simulink model "Aenea_model"  (R2020b)
settings: Solver=FixedStepDiscrete  StartTime=0.0  StopTime=10.0  FixedStep=0.02  RelTol=1e-3
undefined symbols (not defined in the file): attuatore_Amax, attuatore_Amin, attuatore_Emax, attuatore_Emin, attuatore_Rmax, attuatore_Rmin, attuatore_Tmax, attuatore_Tmin, bias, DiscIntNeverNeededParam, interventoA_05, interventoA_1, interventoE_05, interventoE_1, interventoT, inv_A, inv_comp_h, inv_E, inv_R, inv_T, K_AW_B_AP_quota, K_AW_B_becc, K_AW_B_imb, K_AW_B_roll, K_imb_inv, Kd_h_app, Kd_h_flare, Ki_AP_quota_select, Ki_AP_rotta, Ki_AP_vel, Ki_becch, Ki_h_app, Ki_h_cruise, Ki_h_flare, Ki_roll, Kp_AP_quota_hold_h, Kp_AP_quota_hold_l, Kp_AP_quota_select, Kp_AP_rotta, Kp_AP_vel, Kp_becch, Kp_comp_h, Kp_h_app_max, Kp_h_app_min, Kp_h_cruise, Kp_h_flare, Kp_imb, Kp_p, Kp_q, Kp_roll, Kp_Rotta_ATO, Newton, phi_max, phi_min, Q1B, R1B, Raphson, safe_phi, safe_V, Sensor_Offsets ... (+12)
libraries: simulink_extras x37, pid_lib x8, dspsigops x4, arduinolib x3, svdutilitieslib x3, simulink x2, aerolibtransform2sys x2, aerolibtransform2 x2, aerosimlib x2, cstblocks x1
(part 3 of 7)

== system Aenea_model/RADIOCOMANDO/AILERON1 ==
  pwm_aileron_max : Inport
  In1 : Inport  Port=2
  pwm_aileron_min : Inport  Port=3
  Constant8 : Constant  Value=phi_max  OutDataTypeStr=double  SampleTime=-1
  Constant9 : Constant  Value=phi_min  OutDataTypeStr=double  SampleTime=-1
  Divide : Product  Inputs=*/
  Gain : Gain  Gain=-1
  Multiply : Product
  Saturation : Saturate  UpperLimit=phi_max  LowerLimit=phi_min
  Sum : Sum  Inputs=|+-
  Sum1 : Sum  Inputs=|+-
  Sum2 : Sum  Inputs=|+-
  Sum3 : Sum  Inputs=|++
  Out1 : Outport  VectorParamsAs1DForOutWhenUnconnected=off
  wires:
  Divide/1 -> Multiply/1
  Sum/1 -> Divide/1
  In1/1 -> Sum/1
  Constant8/1 -> Sum2/1
  pwm_aileron_min/1 -> Sum1/2, Sum/2
  pwm_aileron_max/1 -> Sum1/1
  Multiply/1 -> Sum3/1
  Sum2/1 -> Multiply/2
  Constant9/1 -> Sum3/2, Sum2/2
  Sum1/1 -> Divide/2
  Sum3/1 -> Gain/1
  Gain/1 -> Saturation/1
  Saturation/1 -> Out1/1

== system Aenea_model/RADIOCOMANDO/ELEVATOR ==
  pwm_elevator_max : Inport
  In1 : Inport  Port=2
  pwm_elevator_min : Inport  Port=3
  Constant8 : Constant  Value=attuatore_Emax  OutDataTypeStr=double  SampleTime=-1
  Constant9 : Constant  Value=attuatore_Emin  OutDataTypeStr=double  SampleTime=-1
  Divide : Product  Inputs=*/
  Multiply : Product
  Sum : Sum  Inputs=|+-
  Sum1 : Sum  Inputs=|+-
  Sum2 : Sum  Inputs=|+-
  Sum3 : Sum  Inputs=|++
  Out1 : Outport  VectorParamsAs1DForOutWhenUnconnected=off
  wires:
  Sum3/1 -> Out1/1
  Multiply/1 -> Sum3/1
  Constant9/1 -> Sum3/2, Sum2/2
  Sum1/1 -> Divide/2
  Sum2/1 -> Multiply/2
  pwm_elevator_min/1 -> Sum1/2, Sum/2
  Constant8/1 -> Sum2/1
  pwm_elevator_max/1 -> Sum1/1
  Divide/1 -> Multiply/1
  In1/1 -> Sum/1
  Sum/1 -> Divide/1

== system Aenea_model/RADIOCOMANDO/ELEVATOR1 ==
  pwm_elevator_max : Inport
  In1 : Inport  Port=2
  pwm_elevator_min : Inport  Port=3
  Constant8 : Constant  Value=theta_max  OutDataTypeStr=double  SampleTime=-1
  Constant9 : Constant  Value=theta_min  OutDataTypeStr=double  SampleTime=-1
  Divide : Product  Inputs=*/
  Gain : Gain
  Multiply : Product
  Saturation : Saturate  UpperLimit=theta_max  LowerLimit=theta_min
  Sum : Sum  Inputs=|+-
  Sum1 : Sum  Inputs=|+-
  Sum2 : Sum  Inputs=|+-
  Sum3 : Sum  Inputs=|++
  Out1 : Outport  VectorParamsAs1DForOutWhenUnconnected=off
  wires:
  Sum3/1 -> Gain/1
  Multiply/1 -> Sum3/1
  Constant9/1 -> Sum3/2, Sum2/2
  Sum1/1 -> Divide/2
  Sum2/1 -> Multiply/2
  pwm_elevator_min/1 -> Sum1/2, Sum/2
  Constant8/1 -> Sum2/1
  pwm_elevator_max/1 -> Sum1/1
  Divide/1 -> Multiply/1
  In1/1 -> Sum/1
  Sum/1 -> Divide/1
  Gain/1 -> Saturation/1
  Saturation/1 -> Out1/1

== system Aenea_model/RADIOCOMANDO/RUDDER ==
  pwm_rudder_max : Inport
  In1 : Inport  Port=2
  pwm_rudder_min : Inport  Port=3
  Constant8 : Constant  Value=attuatore_Rmax  OutDataTypeStr=double  SampleTime=-1
  Constant9 : Constant  Value=attuatore_Rmin  OutDataTypeStr=double  SampleTime=-1
  Divide : Product  Inputs=*/
  Multiply : Product
  Sum1 : Sum  Inputs=|+-
  Sum2 : Sum  Inputs=|+-
  Sum3 : Sum  Inputs=|+-
  Sum4 : Sum  Inputs=|++
  Out1 : Outport  VectorParamsAs1DForOutWhenUnconnected=off
  wires:
  Divide/1 -> Multiply/1
  Sum2/1 -> Divide/2
  pwm_rudder_min/1 -> Sum1/2, Sum2/2
  Sum3/1 -> Multiply/2
  Multiply/1 -> Sum4/1
  Constant9/1 -> Sum4/2, Sum3/2
  Sum1/1 -> Divide/1
  Constant8/1 -> Sum3/1
  pwm_rudder_max/1 -> Sum2/1
  Sum4/1 -> Out1/1
  In1/1 -> Sum1/1

== system Aenea_model/RADIOCOMANDO/THROTTLE ==
  pwm_throttle_max : Inport
  In1 : Inport  Port=2
  pwm_throttle_min : Inport  Port=3
  Divide2 : Product  Inputs=*/
  Multiply1 : Product
  Sum2 : Sum  Inputs=|+-
  Sum3 : Sum  Inputs=|+-
  Sum4 : Sum  Inputs=|+-
  Sum5 : Sum  Inputs=|++
  manetta_massima : Constant  Value=attuatore_Tmax  OutDataTypeStr=double  SampleTime=-1
  manetta_minima : Constant  Value=attuatore_Tmin  OutDataTypeStr=double  SampleTime=-1
  Out1 : Outport  VectorParamsAs1DForOutWhenUnconnected=off
  wires:
  Sum4/1 -> Multiply1/2
  Divide2/1 -> Multiply1/1
  pwm_throttle_max/1 -> Sum3/1
  Sum3/1 -> Divide2/2
  Sum2/1 -> Divide2/1
  manetta_minima/1 -> Sum4/2, Sum5/2
  pwm_throttle_min/1 -> Sum3/2, Sum2/2
  In1/1 -> Sum2/1
  Multiply1/1 -> Sum5/1
  Sum5/1 -> Out1/1
  manetta_massima/1 -> Sum4/1

== system Aenea_model/Servi/AILERON1 ==
  pwm_aileron_max : Inport
  In1 : Inport  Port=2
  pwm-aileron_min : Inport  Port=3
  Constant : Constant  Value=attuatore_Amax  SampleTime=t_AP
  Constant1 : Constant  Value=attuatore_Amin  SampleTime=t_AP
  Divide : Product  Inputs=*/
  Multiply : Product
  Sum : Sum  Inputs=|+-
  Sum1 : Sum  Inputs=|+-
  Sum2 : Sum  Inputs=|+-
  Sum3 : Sum  Inputs=|++
  Out1 : Outport  VectorParamsAs1DForOutWhenUnconnected=off
  wires:
  Sum/1 -> Divide/1
  Constant1/1 -> Sum1/2, Sum/2
  In1/1 -> Sum/1
  Divide/1 -> Multiply/1
  Sum2/1 -> Multiply/2
  pwm-aileron_min/1 -> Sum2/2, Sum3/2
  Multiply/1 -> Sum3/1
  Sum3/1 -> Out1/1
  pwm_aileron_max/1 -> Sum2/1
  Constant/1 -> Sum1/1
  Sum1/1 -> Divide/2

== system Aenea_model/Servi/RUDDER6 ==
  pwm_rudder_max : Inport
  In1 : Inport  Port=2
  "pwm_rudder_min " : Inport  Port=3
  Constant : Constant  Value=attuatore_Rmax  SampleTime=t_AP
  Constant1 : Constant  Value=attuatore_Rmin  SampleTime=t_AP
  Divide : Product  Inputs=*/
  Multiply : Product
  Sum : Sum  Inputs=|+-
  Sum1 : Sum  Inputs=|+-
  Sum2 : Sum  Inputs=|+-
  Sum3 : Sum  Inputs=|++
  Out1 : Outport  VectorParamsAs1DForOutWhenUnconnected=off
  wires:
  Sum/1 -> Divide/1
  Constant1/1 -> Sum1/2, Sum/2
  In1/1 -> Sum/1
  Divide/1 -> Multiply/1
  Sum2/1 -> Multiply/2
  "pwm_rudder_min "/1 -> Sum2/2, Sum3/2
  Multiply/1 -> Sum3/1
  Sum3/1 -> Out1/1
  pwm_rudder_max/1 -> Sum2/1
  Constant/1 -> Sum1/1
  Sum1/1 -> Divide/2

== system Aenea_model/Servi/THROTTLE1 ==
  pwm_throttle_max : Inport
  In1 : Inport  Port=2
  pwm_throttle_min : Inport  Port=3
  Multiply : Product
  Sum : Sum  Inputs=|++  AccumDataTypeStr=int16  OutDataTypeStr=int16
  Sum1 : Sum  Inputs=|+-
  Out1 : Outport  VectorParamsAs1DForOutWhenUnconnected=off
  wires:
  pwm_throttle_min/1 -> Sum/2, Sum1/2
  Sum/1 -> Out1/1
  Multiply/1 -> Sum/1
  pwm_throttle_max/1 -> Sum1/1
  Sum1/1 -> Multiply/2
  In1/1 -> Multiply/1

== system Aenea_model/Servi/elevator ==
  pwm_elevator_max : Inport
  In1 : Inport  Port=2
  pwm_elevator_min : Inport  Port=3
  Constant : Constant  Value=attuatore_Emax  SampleTime=t_AP
  Constant1 : Constant  Value=attuatore_Emin  SampleTime=t_AP
  Divide : Product  Inputs=*/
  Multiply : Product
  Sum : Sum  Inputs=|+-
  Sum1 : Sum  Inputs=|+-
  Sum2 : Sum  Inputs=|+-
  Sum3 : Sum  Inputs=|++
  Out1 : Outport  VectorParamsAs1DForOutWhenUnconnected=off
  wires:
  In1/1 -> Sum/1
  Constant1/1 -> Sum1/2, Sum/2
  Constant/1 -> Sum1/1
  Sum/1 -> Divide/1
  Sum1/1 -> Divide/2
  Divide/1 -> Multiply/1
  pwm_elevator_max/1 -> Sum2/1
  pwm_elevator_min/1 -> Sum2/2, Sum3/2
  Sum2/1 -> Multiply/2
  Multiply/1 -> Sum3/1
  Sum3/1 -> Out1/1

== system Aenea_model/AIR TX/Enable /Chart/sendbyte ==
  note: sostituito con lo stesso blocco della V. R2015a il 29/1/2016
  bt : Inport  OutDataTypeStr=uint8
  n : Inport  Port=2
  f : TriggerPort  TriggerType=function-call  VariantControl=(inherit)
      settings: CopyFcn=Stateflow.SLINSF.SimulinkMan.removeBlockPreDeleteFcn  PreDeleteFcn=Stateflow.SLINSF.SimulinkMan.unsafePredeleteFcn
  Selector : Selector  InputPortWidth=264  IndexOptions=Index vector (port)  Indices=[1 3]  OutputSizes=1
  Serial Transmit : arduinolib/Serial Transmit  Commented=on  portNumber=2  sendmode=write  sendformat=Decimal  floatprecision=2  blockPlatform=arduino
  Terminator : Terminator
  wires:
  Selector/1 -> Terminator/1
  n/1 -> Selector/2
  bt/1 -> Selector/1

== system Aenea_model/AIR TX/If_subsystem/Subsystem ==
  Add : Sum  Inputs=+++
  Add1 : Sum  Inputs=+++
  Add2 : Sum  Inputs=+++
  Constant : Constant  Value=0  SampleTime=0.02
  Constant1 : Constant  Value=0.02  SampleTime=0.02
  Constant2 : Constant  Value=0  SampleTime=t_AP
  Constant3 : Constant  SampleTime=t_AP
  Constant4 : Constant  Value=0  SampleTime=5*t_AP
  Constant5 : Constant  SampleTime=5*t_AP
  Memory : Memory  InitialCondition=-0.02  InheritSampleTime=on
  Memory1 : Memory  InitialCondition=-1  InheritSampleTime=on
  Memory2 : Memory  InitialCondition=-1  InheritSampleTime=on
  Rate Transition : RateTransition  Deterministic=off  OutPortSampleTime=t_AP
  Switch : Switch  Criteria=u2 > Threshold  Threshold=4
  Switch1 : Switch  Criteria=u2 > Threshold  Threshold=9
  H_50 : Outport  VectorParamsAs1DForOutWhenUnconnected=off
  H_10 : Outport  Port=2  VectorParamsAs1DForOutWhenUnconnected=off
  time : Outport  Port=3  VectorParamsAs1DForOutWhenUnconnected=off
  wires:
  Memory1/1 -> Add1/3
  Add2/1 -> Switch1/2, Switch1/3
  Constant4/1 -> Add2/1, Switch1/1
  Constant5/1 -> Add2/2
  Memory2/1 -> Add2/3
  Memory/1 -> Add/3
  Add/1 -> time/1, Memory/1
  Constant/1 -> Add/1
  Constant1/1 -> Add/2
  Constant2/1 -> Add1/1, Switch/1
  Switch/1 -> H_50/1, Memory1/1
  Constant3/1 -> Add1/2
  Add1/1 -> Switch/2, Switch/3
  Switch1/1 -> Rate Transition/1, Memory2/1
  Rate Transition/1 -> H_10/1

== system Aenea_model/AIR TX/Servo/Conversione ==
  Manetta : Inport
  Equilibratore : Inport  Port=2
  Alettoni : Inport  Port=3
  Timone : Inport  Port=4
  Constant2 : Constant  Value=90
  Gain2 : Gain  Gain=100
  Radians to Degrees1 : simulink_extras/Transformations/Radians to Degrees
  Radians to Degrees2 : simulink_extras/Transformations/Radians to Degrees
  Radians to Degrees3 : simulink_extras/Transformations/Radians to Degrees
  Sum : Sum  Inputs=|++
  Sum1 : Sum  Inputs=|++
  Sum2 : Sum  Inputs=|++
  Out1 : Outport  VectorParamsAs1DForOutWhenUnconnected=off
  Out2 : Outport  Port=2  VectorParamsAs1DForOutWhenUnconnected=off
  Out3 : Outport  Port=3  VectorParamsAs1DForOutWhenUnconnected=off
  Out4 : Outport  Port=4  VectorParamsAs1DForOutWhenUnconnected=off
  wires:
  Sum2/1 -> Out4/1
  Timone/1 -> Radians to Degrees3/1
  Sum1/1 -> Out3/1
  Alettoni/1 -> Radians to Degrees2/1
  Sum/1 -> Out2/1
  Equilibratore/1 -> Radians to Degrees1/1
  Gain2/1 -> Out1/1
  Manetta/1 -> Gain2/1
  Constant2/1 -> Sum2/2, Sum1/2, Sum/2
  Radians to Degrees3/1 -> Sum2/1
  Radians to Degrees2/1 -> Sum1/1
  Radians to Degrees1/1 -> Sum/1

== system Aenea_model/AIR TX/VFR/wrapTo360 ==
  In1 : Inport
  Abs : Abs
  Constant2 : Constant  Value=360
  Sum : Sum  Inputs=-+|
  Switch2 : Switch  Criteria=u2 > Threshold
  Out1 : Outport  VectorParamsAs1DForOutWhenUnconnected=off
  wires:
  Sum/1 -> Switch2/3
  Abs/1 -> Sum/1
  Constant2/1 -> Sum/2
  In1/1 -> Switch2/1, Switch2/2, Abs/1
  Switch2/1 -> Out1/1

== system Aenea_model/AUTOPILOTA/AUTOPILOTI1/CONTROLLORE DI QUOTA ==
  Sensori : Inport
  Riferimenti : Inport  Port=2
  Parametri Sistema di Controllo : Inport  Port=3
  Ato : Inport  Port=4
  traking_theta : Inport  Port=5
  Abs : Abs
  Bus Selector : BusSelector  OutputSignals=Kp_AP_quota_hold
  Bus Selector2 : BusSelector  OutputSignals=RC,Alt,Tas,theta
  Bus Selector3 : BusSelector  OutputSignals=QUOTA,RC,landing_selector
  Controllore di RC1 : Subsystem
  Kp : Product  RndMeth=Zero
  SELEZIONE MODALITA' HOLD/SELECT : Stateflow chart  TreatAsAtomicUnit=on
  "Saturazione RC " : Subsystem
  Sum1 : Sum  Inputs=+-
  Switch HOLD/SELECT : MultiPortSwitch  DataPortOrder=Zero-based contiguous  Inputs=2  zeroidx=on
  theta_rif : Outport  VectorParamsAs1DForOutWhenUnconnected=off
  tag scope: RC=global, RC_rif=global, V=global, h=global, h_rif=global, landing_selector=global, parametri_est=global, theta=global
  wires:
  Sensori/1 -> Bus Selector2/1
  Riferimenti/1 -> Bus Selector3/1
  Parametri Sistema di Controllo/1 -> [parametri_est]
  Bus Selector2/1 -> [RC]  "<RC>"
  Bus Selector2/2 -> [h]  "<Alt>"
  Bus Selector2/3 -> [V]  "<Tas>"
  Bus Selector2/4 -> [theta]  "<theta>"
  Bus Selector3/1 -> [h_rif]  "<QUOTA>"
  Bus Selector3/2 -> [RC_rif]  "<RC>"
  [V] -> "Saturazione RC "/1(V)
  Sum1/1 -> Abs/1, Kp/1  "errore_h"
  [h_rif] -> Sum1/1
  [h] -> Sum1/2
  Abs/1 -> SELEZIONE MODALITA' HOLD/SELECT/1(deltah)
  Kp/1 -> Switch HOLD/SELECT/2
  [RC_rif] -> Switch HOLD/SELECT/3
  SELEZIONE MODALITA' HOLD/SELECT/1(mod) -> Switch HOLD/SELECT/1, Controllore di RC1/7(saturation)
  [parametri_est] -> Bus Selector/1
  Bus Selector/1 -> Kp/2  "<Kp_AP_quota_hold>"
  Switch HOLD/SELECT/1 -> "Saturazione RC "/2(RC)
  Bus Selector3/3 -> [landing_selector]  "<landing_selector>"
  [h] -> Controllore di RC1/2(h)
  [h_rif] -> Controllore di RC1/1(h_rif)
  [landing_selector] -> Controllore di RC1/4(landing_selector)
  Ato/1 -> Controllore di RC1/3("Ato ")
  Controllore di RC1/1(theta_rif) -> theta_rif/1
  [RC] -> Controllore di RC1/6(RC)
  "Saturazione RC "/1(RC_verficata) -> Controllore di RC1/5(RC_rif_cruise)
  [RC_rif] -> Controllore di RC1/8("RC_al ")
  traking_theta/1 -> Controllore di RC1/9(traking)
  [V] -> Controllore di RC1/10(tas)

== system Aenea_model/AUTOPILOTA/AUTOPILOTI1/CONTROLLORE DI ROTTA ==
  Riferimenti : Inport
  Sensori : Inport  Port=2
  Parametri Sistema di Controllo : Inport  Port=3
  "switch alettoni " : Inport  Port=4
  track_phi : Inport  Port=5
  Switch_ATO : Inport  Port=6
  ATO : Subsystem
  Bus Selector1 : BusSelector  OutputSignals=ROTTA
  Bus Selector3 : BusSelector  OutputSignals=Kp_AP_rotta,Ki_AP_rotta
  Bus Selector4 : BusSelector  OutputSignals=heading,horiz_speed,Tas,phi,Alt,psi
  Constant : Constant  Value=70
  Constant2 : Constant  Value=Ki_AP_rotta
  PID Controller1 : pid_lib/PID Controller  Controller=PID  Form=Parallel  TimeDomain=Discrete-time  UseExternalTs=off  SampleTime=-1  IntegratorMethod=Forward Euler  FilterMethod=Forward Euler  ControllerParametersSource=external  P=1  I=1  D=0  UseFilter=on  N=100  TunerSelectOption=Transfer Function Based (PID Tuner App)  InitialConditionSource=internal  InitialConditionForIntegrator=0  InitialConditionForFilter=0  DifferentiatorICPrevScaledInput=0  ExternalReset=none  TrackingMode=on  Kt=1  LimitOutput=on  SatLimitsSource=internal  UpperSaturationLimit=0.7854  LowerSaturationLimit=-0.7854  LinearizeAsGain=on  AntiWindupMode=clamping  Kb=0.1  POutMin=[]  POutMax=[]  IOutMin=[]  IOutMax=[]  DOutMin=[]  DOutMax=[]  NOutMin=[]  NOutMax=[]  SumOutMin=[]  SumOutMax=[]  SaturationOutMin=[]  SaturationOutMax=[]  PParamMin=[]  PParamMax=[]  IParamMin=[]  IParamMax=[]  DParamMin=[]  DParamMax=[]  NParamMin=[]  NParamMax=[]  KbParamMin=[]  KbParamMax=[]  KtParamMin=[]  KtParamMax=[]  KbOutMin=[]  KbOutMax=[]  KtOutMin=[]  KtOutMax=[]  IntegratorOutMin=[]  IntegratorOutMax=[]  FilterOutMin=[]  FilterOutMax=[]  SumI1OutMin=[]  SumI1OutMax=[]  SumI2OutMin=[]  SumI2OutMax=[]  SumI3OutMin=[]  SumI3OutMax=[]  SumI4OutMin=[]  SumI4OutMax=[]  SumDOutMin=[]  SumDOutMax=[]  DifferentiatorOutMin=[]  DifferentiatorOutMax=[]  FilterDiffOutCoefMin=[]  FilterDiffOutCoefMax=[]  ReciprocalOutMin=[]  ReciprocalOutMax=[]  SumDenOutMin=[]  SumDenOutMax=[]  SumNumOutMin=[]  SumNumOutMax=[]  DivideOutMin=[]  DivideOutMax=[]  UdiffTsProdOutMin=[]  UdiffTsProdOutMax=[]  NTsProdOutMin=[]  NTsProdOutMax=[]  UintegralTsProdOutMin=[]  UintegralTsProdOutMax=[]  UngainTsProdOutMin=[]  UngainTsProdOutMax=[]  IntegratorContinuousStateAttributes=''  IntegratorStateMustResolveToSignalObject=off  IntegratorRTWStateStorageClass=Auto  FilterContinuousStateAttributes=''  FilterStateMustResolveToSignalObject=off  FilterRTWStateStorageClass=Auto  ParallelPVariant=ExternalParameters  IdealPVariant=Disabled  IVariant=ExternalParameters  DVariant=ExternalParameters  IntegratorVariant=Discrete  SatVariant=Enabled  AWVariant=DiscClampingParallel  PCopyVariant=Disabled  TRVariant=Enabled  FdbkBlocksVariant=Forward  IdealPFdbkVariant=Disabled  SatFdbkVariant=Disabled  DerivativeFilterVariant=ForwardEulerFilter  NVariant=ExternalParameters  NCopyVariant=Disabled  FilterICVariant=InternalICsFilter  IntegratorICVariant=InternalICs  ExternalResetVariant=Disabled  TRSumVariant=TrackingMode  SumFdbkVariant=Disabled  SumVariant=Sum_PID  TsampFilterVariant=InternalTs  TsampNgainVariant=Passthrough  TsampIntegralVariant=Passthrough  ExternalSaturationOutDataTypeStr=Inherit: Same as second input
  Switch : Switch  Criteria=u2 > Threshold  Threshold=5
  Switch auto-manual : MultiPortSwitch  DataPortOrder=Zero-based contiguous  Inputs=2  zeroidx=on
  "calcolo errore Psi " : Subsystem
  phi_rif : Outport  VectorParamsAs1DForOutWhenUnconnected=off
  tag scope: Vel=global
  wires:
  Bus Selector1/1 -> "calcolo errore Psi "/1(psi_ref (°))  "<ROTTA>"
  Sensori/1 -> Bus Selector4/1
  Riferimenti/1 -> Bus Selector1/1
  Bus Selector4/1 -> [heading]  "<heading>"
  Bus Selector4/3 -> [Vel]  "<Tas>"
  [rotta_mis] -> "calcolo errore Psi "/2(psi (rad))
  Bus Selector4/4 -> [phi]  "<phi>"
  Parametri Sistema di Controllo/1 -> Bus Selector3/1
  "calcolo errore Psi "/1(psi_err) -> PID Controller1/1
  Constant/1 -> PID Controller1/5
  PID Controller1/1 -> Switch auto-manual/3
  Bus Selector4/5 -> [Alt]  "<Alt>"
  Bus Selector3/2 -> ATO/4(In4)  "<Ki_AP_rotta>"
  Bus Selector3/1 -> ATO/1(In1)  "<Kp_AP_rotta>"
  Constant2/1 -> PID Controller1/3
  "switch alettoni "/1 -> Switch auto-manual/1
  Bus Selector4/6 -> [psi]  "<psi>"
  ? -> [V_]  "<v>"
  [V_] -> Switch/2
  [heading] -> Switch/1
  [psi] -> Switch/3
  Switch/1 -> [rotta_mis]
  Switch auto-manual/1 -> phi_rif/1
  track_phi/1 -> PID Controller1/6
  ATO/1(Out1) -> PID Controller1/2
  ATO/2(Out2) -> PID Controller1/4
  [Alt] -> ATO/3(In3)
  Switch_ATO/1 -> [Switch_ATO]
  [Switch_ATO] -> ATO/2(In2)
  [phi] -> Switch auto-manual/2

== system Aenea_model/AUTOPILOTA/AUTOPILOTI1/CONTROLLORE DI VELOCITA' ==
  note: CANALE DI
      |  VELOCITA'
  Sensori : Inport
  Riferimenti : Inport  Port=2
  Parametri Sistema di Controllo : Inport  Port=3
  switch_manetta : Inport  Port=4
  comandi : Inport  Port=5
  Switch_AL : Inport  Port=6
  manetta_track : Inport  Port=7
  Bus Selector : BusSelector  OutputSignals=VELOCITA,QUOTA
  Bus Selector1 : BusSelector  OutputSignals=Tas,Alt,quota_lidar
  Bus Selector2 : BusSelector  OutputSignals=Kp_AP_vel,Ki_AP_vel
  Bus Selector3 : BusSelector  OutputSignals=Manual Throttle
  PID Controller : pid_lib/PID Controller  Controller=PI  Form=Parallel  TimeDomain=Discrete-time  UseExternalTs=off  SampleTime=-1  IntegratorMethod=Forward Euler  FilterMethod=Forward Euler  ControllerParametersSource=external  P=1  I=1  D=0  UseFilter=on  N=100  TunerSelectOption=Transfer Function Based (PID Tuner App)  InitialConditionSource=internal  InitialConditionForIntegrator=0  InitialConditionForFilter=0  DifferentiatorICPrevScaledInput=0  ExternalReset=none  TrackingMode=on  Kt=1  LimitOutput=on  SatLimitsSource=internal  UpperSaturationLimit=attuatore_Tmax  LowerSaturationLimit=attuatore_Tmin  LinearizeAsGain=on  AntiWindupMode=clamping  Kb=1  POutMin=[]  POutMax=[]  IOutMin=[]  IOutMax=[]  DOutMin=[]  DOutMax=[]  NOutMin=[]  NOutMax=[]  SumOutMin=[]  SumOutMax=[]  SaturationOutMin=[]  SaturationOutMax=[]  PParamMin=[]  PParamMax=[]  IParamMin=[]  IParamMax=[]  DParamMin=[]  DParamMax=[]  NParamMin=[]  NParamMax=[]  KbParamMin=[]  KbParamMax=[]  KtParamMin=[]  KtParamMax=[]  KbOutMin=[]  KbOutMax=[]  KtOutMin=[]  KtOutMax=[]  IntegratorOutMin=[]  IntegratorOutMax=[]  FilterOutMin=[]  FilterOutMax=[]  SumI1OutMin=[]  SumI1OutMax=[]  SumI2OutMin=[]  SumI2OutMax=[]  SumI3OutMin=[]  SumI3OutMax=[]  SumI4OutMin=[]  SumI4OutMax=[]  SumDOutMin=[]  SumDOutMax=[]  DifferentiatorOutMin=[]  DifferentiatorOutMax=[]  FilterDiffOutCoefMin=[]  FilterDiffOutCoefMax=[]  ReciprocalOutMin=[]  ReciprocalOutMax=[]  SumDenOutMin=[]  SumDenOutMax=[]  SumNumOutMin=[]  SumNumOutMax=[]  DivideOutMin=[]  DivideOutMax=[]  UdiffTsProdOutMin=[]  UdiffTsProdOutMax=[]  NTsProdOutMin=[]  NTsProdOutMax=[]  UintegralTsProdOutMin=[]  UintegralTsProdOutMax=[]  UngainTsProdOutMin=[]  UngainTsProdOutMax=[]  IntegratorContinuousStateAttributes=''  IntegratorStateMustResolveToSignalObject=off  IntegratorRTWStateStorageClass=Auto  FilterContinuousStateAttributes=''  FilterStateMustResolveToSignalObject=off  FilterRTWStateStorageClass=Auto  ParallelPVariant=ExternalParameters  IdealPVariant=Disabled  IVariant=ExternalParameters  DVariant=Disabled  IntegratorVariant=Discrete  SatVariant=Enabled  AWVariant=DiscClampingParallel  PCopyVariant=Disabled  TRVariant=Enabled  FdbkBlocksVariant=Forward  IdealPFdbkVariant=Disabled  SatFdbkVariant=Disabled  DerivativeFilterVariant=Disabled  NVariant=Disabled  NCopyVariant=Disabled_SignalSpec  FilterICVariant=Disabled  IntegratorICVariant=InternalICs  ExternalResetVariant=Disabled  TRSumVariant=TrackingMode  SumFdbkVariant=Disabled  SumVariant=Sum_PI  TsampFilterVariant=InternalTs  TsampNgainVariant=Passthrough  TsampIntegralVariant=Passthrough  ExternalSaturationOutDataTypeStr=Inherit: Same as second input
  Smooth Switch : Subsystem
  Sum3 : Sum  Inputs=-+
  throttle - landing : Subsystem
  Riferimento Manetta : Outport  VectorParamsAs1DForOutWhenUnconnected=off
  wires:
  Sensori/1 -> Bus Selector1/1
  Riferimenti/1 -> Bus Selector/1
  Bus Selector/1 -> Sum3/2  "<VELOCITA>"
  Bus Selector1/1 -> [Tas], Sum3/1  "<Tas>"
  comandi/1 -> Bus Selector3/1
  Sum3/1 -> PID Controller/1  "e"
  switch_manetta/1 -> [switch_manetta]
  Bus Selector1/2 -> [Alt]  "<Alt>"
  Parametri Sistema di Controllo/1 -> Bus Selector2/1
  Bus Selector2/1 -> PID Controller/2  "<Kp_AP_vel>"
  Bus Selector2/2 -> PID Controller/3  "<Ki_AP_vel>"
  Bus Selector3/1 -> [Manual_Throttle]  "<Manual Throttle>"
  [quota_al_ref] -> throttle - landing/3(Alt)
  Switch_AL/1 -> throttle - landing/1(AL)
  throttle - landing/1(Out1) -> Riferimento Manetta/1
  Bus Selector1/3 -> [quota_lidar]  "<quota_lidar>"
  Bus Selector/2 -> [quota_al_ref]  "<QUOTA>"
  manetta_track/1 -> PID Controller/4
  PID Controller/1 -> Smooth Switch/3(manetta_controllo)
  [switch_manetta] -> Smooth Switch/1(switch_manetta)
  Smooth Switch/1(Out1) -> throttle - landing/2(In2)
  [Manual_Throttle] -> Smooth Switch/2(manetta_manuale)

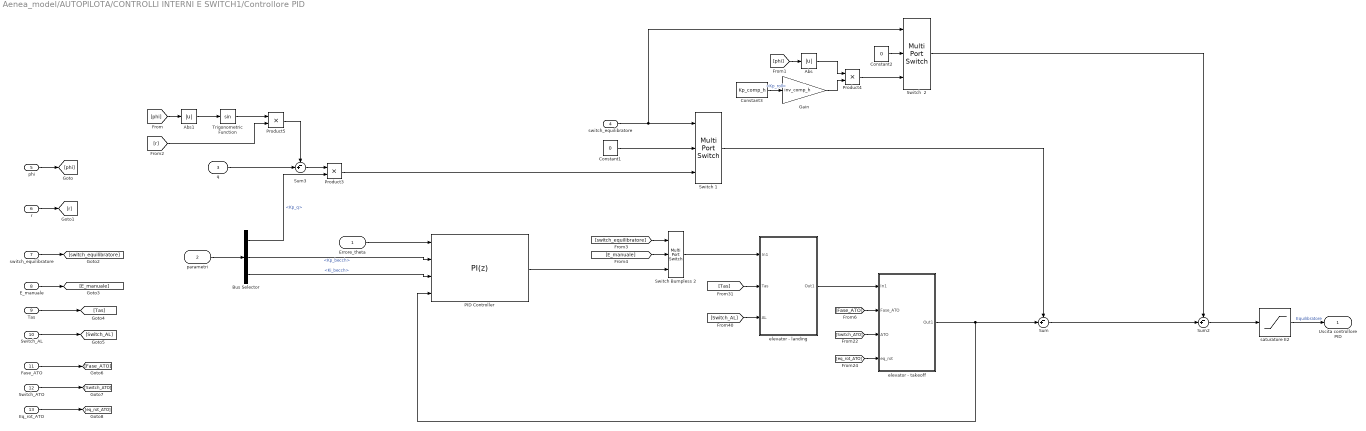
== system Aenea_model/AUTOPILOTA/CONTROLLI INTERNI E SWITCH1/Controllore PID ==
  Errore_theta : Inport
  parametri : Inport  Port=2
  "q " : Inport  Port=3
  "switch_equilibratore " : Inport  Port=4
  "phi " : Inport  Port=5
  r : Inport  Port=6
  switch_equilibratore : Inport  Port=7
  E_manuale : Inport  Port=8
  Tas : Inport  Port=9
  Switch_AL : Inport  Port=10
  Fase_ATO : Inport  Port=11
  Switch_ATO : Inport  Port=12
  Eq_rot_ATO : Inport  Port=13
  Abs : Abs
  Abs1 : Abs
  Bus Selector : BusSelector  OutputSignals=Kp_q,Kp_becch,Ki_becch
  Constant1 : Constant  Value=0  SampleTime=0.02
  Constant2 : Constant  Value=0  SampleTime=0.02
  Constant3 : Constant  Value=Kp_comp_h  SampleTime=0.02
  Gain : Gain  Gain=inv_comp_h
  PID Controller : pid_lib/PID Controller  Controller=PI  Form=Parallel  TimeDomain=Discrete-time  UseExternalTs=off  SampleTime=-1  IntegratorMethod=Forward Euler  FilterMethod=Forward Euler  ControllerParametersSource=external  P=1  I=1  D=1  UseFilter=off  N=100  TunerSelectOption=Transfer Function Based (PID Tuner App)  InitialConditionSource=internal  InitialConditionForIntegrator=0  InitialConditionForFilter=0  DifferentiatorICPrevScaledInput=0  ExternalReset=none  TrackingMode=on  Kt=1  LimitOutput=on  SatLimitsSource=internal  UpperSaturationLimit=attuatore_Emax  LowerSaturationLimit=attuatore_Emin  LinearizeAsGain=on  AntiWindupMode=back-calculation  Kb=1  POutMin=[]  POutMax=[]  IOutMin=[]  IOutMax=[]  DOutMin=[]  DOutMax=[]  NOutMin=[]  NOutMax=[]  SumOutMin=[]  SumOutMax=[]  SaturationOutMin=[]  SaturationOutMax=[]  PParamMin=[]  PParamMax=[]  IParamMin=[]  IParamMax=[]  DParamMin=[]  DParamMax=[]  NParamMin=[]  NParamMax=[]  KbParamMin=[]  KbParamMax=[]  KtParamMin=[]  KtParamMax=[]  KbOutMin=[]  KbOutMax=[]  KtOutMin=[]  KtOutMax=[]  IntegratorOutMin=[]  IntegratorOutMax=[]  FilterOutMin=[]  FilterOutMax=[]  SumI1OutMin=[]  SumI1OutMax=[]  SumI2OutMin=[]  SumI2OutMax=[]  SumI3OutMin=[]  SumI3OutMax=[]  SumI4OutMin=[]  SumI4OutMax=[]  SumDOutMin=[]  SumDOutMax=[]  DifferentiatorOutMin=[]  DifferentiatorOutMax=[]  FilterDiffOutCoefMin=[]  FilterDiffOutCoefMax=[]  ReciprocalOutMin=[]  ReciprocalOutMax=[]  SumDenOutMin=[]  SumDenOutMax=[]  SumNumOutMin=[]  SumNumOutMax=[]  DivideOutMin=[]  DivideOutMax=[]  UdiffTsProdOutMin=[]  UdiffTsProdOutMax=[]  NTsProdOutMin=[]  NTsProdOutMax=[]  UintegralTsProdOutMin=[]  UintegralTsProdOutMax=[]  UngainTsProdOutMin=[]  UngainTsProdOutMax=[]  IntegratorContinuousStateAttributes=''  IntegratorStateMustResolveToSignalObject=off  IntegratorRTWStateStorageClass=Auto  FilterContinuousStateAttributes=''  FilterStateMustResolveToSignalObject=off  FilterRTWStateStorageClass=Auto  ParallelPVariant=ExternalParameters  IdealPVariant=Disabled  IVariant=ExternalParameters  DVariant=Disabled  IntegratorVariant=Discrete  SatVariant=Enabled  AWVariant=BackCalculation  PCopyVariant=Disabled  TRVariant=Enabled  FdbkBlocksVariant=Forward  IdealPFdbkVariant=Disabled  SatFdbkVariant=Disabled  DerivativeFilterVariant=Disabled  NVariant=Disabled  NCopyVariant=Disabled_SignalSpec  FilterICVariant=Disabled  IntegratorICVariant=InternalICs  ExternalResetVariant=Disabled  TRSumVariant=TrackingMode  SumFdbkVariant=Disabled  SumVariant=Sum_PI  TsampFilterVariant=InternalTs  TsampNgainVariant=Passthrough  TsampIntegralVariant=Passthrough  ExternalSaturationOutDataTypeStr=Inherit: Same as second input
  Product3 : Product  RndMeth=Zero
  Product4 : Product  RndMeth=Zero
  Product5 : Product  RndMeth=Zero
  Sum : Sum  Inputs=-+|
  Sum2 : Sum  Inputs=-+|
  Sum3 : Sum  Inputs=-+|
  Switch  2 : MultiPortSwitch  DataPortOrder=Zero-based contiguous  Inputs=2  zeroidx=on
  Switch 1 : MultiPortSwitch  DataPortOrder=Zero-based contiguous  Inputs=2  zeroidx=on
  Switch Bumpless 2 : MultiPortSwitch  DataPortOrder=Zero-based contiguous  Inputs=2  zeroidx=on
  Trigonometric Function : Trigonometry
  elevator - landing : Subsystem
  elevator - takeoff : Subsystem
  saturatore E2 : Saturate  UpperLimit=attuatore_Emax  LowerLimit=attuatore_Emin
  Uscita controllore PID : Outport  VectorParamsAs1DForOutWhenUnconnected=off
  wires:
  Errore_theta/1 -> PID Controller/1
  parametri/1 -> Bus Selector/1
  Bus Selector/2 -> PID Controller/2  "<Kp_becch>"
  Bus Selector/3 -> PID Controller/3  "<Ki_becch>"
  Bus Selector/1 -> Product3/2  "<Kp_q>"
  Switch 1/1 -> Sum/1
  Product3/1 -> Switch 1/3
  Constant1/1 -> Switch 1/2
  elevator - takeoff/1(Out1) -> PID Controller/4, Sum/2
  Sum2/1 -> saturatore E2/1
  [phi] -> Abs/1
  Switch  2/1 -> Sum2/1
  Product4/1 -> Switch  2/3
  Constant2/1 -> Switch  2/2
  "switch_equilibratore "/1 -> Switch  2/1, Switch 1/1
  Abs/1 -> Product4/1
  [phi] -> Abs1/1
  Abs1/1 -> Trigonometric Function/1
  "phi "/1 -> [phi]
  r/1 -> [r]
  Trigonometric Function/1 -> Product5/1
  [r] -> Product5/2
  "q "/1 -> Sum3/2
  Sum3/1 -> Product3/1
  Product5/1 -> Sum3/1
  Sum/1 -> Sum2/2
  Switch Bumpless 2/1 -> elevator - landing/1(In1)
  Gain/1 -> Product4/2
  [Tas] -> elevator - landing/2(Tas)
  [Switch_AL] -> elevator - landing/3(AL)
  [Switch_ATO] -> elevator - takeoff/3(ATO)
  [Fase_ATO] -> elevator - takeoff/2(Fase_ATO)
  [eq_rot_ATO] -> elevator - takeoff/4(eq_rot)
  elevator - landing/1(Out1) -> elevator - takeoff/1(In1)
  [E_manuale] -> Switch Bumpless 2/2
  PID Controller/1 -> Switch Bumpless 2/3
  [switch_equilibratore] -> Switch Bumpless 2/1
  switch_equilibratore/1 -> [switch_equilibratore]
  E_manuale/1 -> [E_manuale]
  Tas/1 -> [Tas]
  Switch_AL/1 -> [Switch_AL]
  Fase_ATO/1 -> [Fase_ATO]
  Switch_ATO/1 -> [Switch_ATO]
  Eq_rot_ATO/1 -> [eq_rot_ATO]
  saturatore E2/1 -> Uscita controllore PID/1  "Equilibratore"
  Constant3/1 -> Gain/1  "<Kp_roll>"

== system Aenea_model/AUTOPILOTA/CONTROLLI INTERNI E SWITCH1/Controllore PID1 ==
  Err_Trk : Inport
  Errore_phi : Inport  Port=2
  parametri : Inport  Port=3
  "p " : Inport  Port=4
  "switch_alettoni " : Inport  Port=5
  Fase_ATO : Inport  Port=6
  Bus Selector : BusSelector  OutputSignals=Kp_p,Kp_roll,Ki_roll
  Constant1 : Constant  Value=0  SampleTime=0.02
  Constant3 : Constant  Value=2
  PID Controller : pid_lib/PID Controller  Controller=PI  Form=Parallel  TimeDomain=Discrete-time  UseExternalTs=off  SampleTime=0.02  IntegratorMethod=Forward Euler  FilterMethod=Forward Euler  ControllerParametersSource=external  P=1  I=1  D=0  UseFilter=on  N=100  TunerSelectOption=Transfer Function Based (PID Tuner App)  InitialConditionSource=internal  InitialConditionForIntegrator=0  InitialConditionForFilter=0  DifferentiatorICPrevScaledInput=0  ExternalReset=rising  TrackingMode=on  Kt=1  LimitOutput=on  SatLimitsSource=internal  UpperSaturationLimit=attuatore_Amax  LowerSaturationLimit=attuatore_Amin  LinearizeAsGain=on  AntiWindupMode=back-calculation  Kb=0.5  POutMin=[]  POutMax=[]  IOutMin=[]  IOutMax=[]  DOutMin=[]  DOutMax=[]  NOutMin=[]  NOutMax=[]  SumOutMin=[]  SumOutMax=[]  SaturationOutMin=[]  SaturationOutMax=[]  PParamMin=[]  PParamMax=[]  IParamMin=[]  IParamMax=[]  DParamMin=[]  DParamMax=[]  NParamMin=[]  NParamMax=[]  KbParamMin=[]  KbParamMax=[]  KtParamMin=[]  KtParamMax=[]  KbOutMin=[]  KbOutMax=[]  KtOutMin=[]  KtOutMax=[]  IntegratorOutMin=[]  IntegratorOutMax=[]  FilterOutMin=[]  FilterOutMax=[]  SumI1OutMin=[]  SumI1OutMax=[]  SumI2OutMin=[]  SumI2OutMax=[]  SumI3OutMin=[]  SumI3OutMax=[]  SumI4OutMin=[]  SumI4OutMax=[]  SumDOutMin=[]  SumDOutMax=[]  DifferentiatorOutMin=[]  DifferentiatorOutMax=[]  FilterDiffOutCoefMin=[]  FilterDiffOutCoefMax=[]  ReciprocalOutMin=[]  ReciprocalOutMax=[]  SumDenOutMin=[]  SumDenOutMax=[]  SumNumOutMin=[]  SumNumOutMax=[]  DivideOutMin=[]  DivideOutMax=[]  UdiffTsProdOutMin=[]  UdiffTsProdOutMax=[]  NTsProdOutMin=[]  NTsProdOutMax=[]  UintegralTsProdOutMin=[]  UintegralTsProdOutMax=[]  UngainTsProdOutMin=[]  UngainTsProdOutMax=[]  IntegratorContinuousStateAttributes=''  IntegratorStateMustResolveToSignalObject=off  IntegratorRTWStateStorageClass=Auto  FilterContinuousStateAttributes=''  FilterStateMustResolveToSignalObject=off  FilterRTWStateStorageClass=Auto  ParallelPVariant=ExternalParameters  IdealPVariant=Disabled  IVariant=ExternalParameters  DVariant=Disabled  IntegratorVariant=Discrete  SatVariant=Enabled  AWVariant=BackCalculation  PCopyVariant=Disabled  TRVariant=Enabled  FdbkBlocksVariant=Forward  IdealPFdbkVariant=Disabled  SatFdbkVariant=Disabled  DerivativeFilterVariant=Disabled  NVariant=Disabled  NCopyVariant=Disabled_SignalSpec  FilterICVariant=Disabled  IntegratorICVariant=InternalICs  ExternalResetVariant=ExternalReset  TRSumVariant=TrackingMode  SumFdbkVariant=Disabled  SumVariant=Sum_PI  TsampFilterVariant=InternalTs  TsampNgainVariant=Passthrough  TsampIntegralVariant=Passthrough  ExternalSaturationOutDataTypeStr=Inherit: Same as second input
  Product3 : Product  RndMeth=Zero
  Sum : Sum  Inputs=|+-
  Sum2 : Sum  Inputs=-+|
  Switch Bumpless 1 : MultiPortSwitch  DataPortOrder=Zero-based contiguous  Inputs=2  zeroidx=on
  Uscita controllore PID : Outport  VectorParamsAs1DForOutWhenUnconnected=off
  wires:
  Errore_phi/1 -> PID Controller/1
  parametri/1 -> Bus Selector/1
  Bus Selector/2 -> PID Controller/2  "<Kp_roll>"
  Bus Selector/3 -> PID Controller/3  "<Ki_roll>"
  "p "/1 -> Product3/1
  Switch Bumpless 1/1 -> Sum2/1
  Product3/1 -> Switch Bumpless 1/3
  "switch_alettoni "/1 -> Switch Bumpless 1/1
  Constant1/1 -> Switch Bumpless 1/2
  Bus Selector/1 -> Product3/2  "<Kp_p>"
  Sum2/1 -> Uscita controllore PID/1
  PID Controller/1 -> Sum2/2
  Err_Trk/1 -> PID Controller/5
  Fase_ATO/1 -> Sum/1
  Constant3/1 -> Sum/2
  Sum/1 -> PID Controller/4

== system Aenea_model/AUTOPILOTA/CONTROLLI INTERNI E SWITCH1/Filtro Washout1 ==
  In : Inport
  Discrete Washout Filter : DiscreteTransferFcn  Numerator=[ 1 -1]  Denominator=[1 -0.995]  SampleTime=t_AP
  Discrete Washout Filter1 : DiscreteTransferFcn  Commented=on  Numerator=[1.234 -1.234]  Denominator=[1 -0.995]  SampleTime=tsamp
  Out : Outport  VectorParamsAs1DForOutWhenUnconnected=off
  wires:
  In/1 -> Discrete Washout Filter/1
  Discrete Washout Filter/1 -> Out/1

== system Aenea_model/AUTOPILOTA/CONTROLLI INTERNI E SWITCH1/manetta - takeoff ==
  note: Quando verra caricato sull'autopilota bisogna modificare il limite del saturatore e metterlo ad 1
  In1 : Inport
  Fase_ATO : Inport  Port=2
  ATO : Inport  Port=3
  manetta_ref_ATO : Inport  Port=4
  Constant4 : Constant  Value=0
  Constant7 : Constant  Value=10
  Constant8 : Constant
  Discrete-Time Integrator : DiscreteIntegrator  gainval=0.015  ExternalReset=rising  SampleTime=-1  LimitOutput=on  UpperSaturationLimit=0.6  LowerSaturationLimit=0  ICPrevOutput=DiscIntNeverNeededParam  ICPrevScaledInput=DiscIntNeverNeededParam
  Multiport Switch1 : MultiPortSwitch  DataPortOrder=Zero-based contiguous  Inputs=2  zeroidx=on
  Sum : Sum  Inputs=|+-
  Switch Bumpless 1 : MultiPortSwitch  DataPortOrder=Zero-based contiguous  Inputs=5  zeroidx=on
  Out1 : Outport  VectorParamsAs1DForOutWhenUnconnected=off
  wires:
  Discrete-Time Integrator/1 -> Switch Bumpless 1/4
  Constant7/1 -> Discrete-Time Integrator/1
  Constant8/1 -> Sum/2
  manetta_ref_ATO/1 -> Switch Bumpless 1/3
  Constant4/1 -> Switch Bumpless 1/2
  ATO/1 -> Multiport Switch1/1
  Switch Bumpless 1/1 -> Multiport Switch1/3
  Sum/1 -> Discrete-Time Integrator/2
  In1/1 -> Multiport Switch1/2, Switch Bumpless 1/5, Switch Bumpless 1/6  "Manetta"
  Fase_ATO/1 -> Switch Bumpless 1/1, Sum/1
  Multiport Switch1/1 -> Out1/1  "Manetta"

== system Aenea_model/AUTOPILOTA/GESTIONE AUTOPILOTI1/Interruttore_Intervento ==
  note: Quando si preme il pulsante per il test dell'intervento pilota su QGC int_sw_intervento = 1 e si attiva l'Enabled Subsystem, quando si riva in manual int_sw_intervento torna a zero e il subsystem non si attiva. Inoltre contemporaneamente ogni volta che int_sw_intervento da 0 passa a 1 si attiva anche il Resettable Subsystem che resetta il clock che altrimenti continuerebbe a contare e non permetterebbe di rifare il test una seconda volta dato che L'Enable Subsystem restituirebbe 0.
  note: Quando è attivo manda un 1 per due secondi e poi 0.
  int_sw_intervento : Inport
  Display : Display
  Display1 : Display
  Enabled Subsystem : Subsystem  TreatAsAtomicUnit=on
  Resettable Subsystem : Subsystem  TreatAsAtomicUnit=on
  1/0 : Outport  VectorParamsAs1DForOutWhenUnconnected=off
  wires:
  int_sw_intervento/1 -> Resettable Subsystem/Reset, Enabled Subsystem/Enable, Display1/1
  Enabled Subsystem/1(1/0) -> Display/1, 1/0/1
  Resettable Subsystem/1(Time) -> Enabled Subsystem/1(Time)

== system Aenea_model/AUTOPILOTA/GESTIONE AUTOPILOTI1/Interruttore_Safe ==
  note: Quando si preme il pulsante per il test del SAFE su QGC int_sw_safe = 1 e si attiva l'Enabled Subsystem, quando si riva in manual int_sw_safe torna a zero e il subsystem non si attiva. Inoltre contemporaneamente ogni volta che int_sw_sefe da 0 passa
      | a 1 si attiva anche il Resettable Subsystem che resetta il clock che altrimenti continuerebbe a contare e non permetterebbe di rifare il test una seconda volta dato che L'Enable Subsystem restituirebbe 0.
  note: Quando è attivo manda un 1 per due secondi e poi 0.
  int_sw_safe : Inport
  Enabled Subsystem : Subsystem  TreatAsAtomicUnit=on
  Resettable Subsystem : Subsystem  TreatAsAtomicUnit=on
  1/0 : Outport  VectorParamsAs1DForOutWhenUnconnected=off
  wires:
  int_sw_safe/1 -> Resettable Subsystem/Reset, Enabled Subsystem/Enable
  Enabled Subsystem/1(1/0) -> 1/0/1
  Resettable Subsystem/1(Time) -> Enabled Subsystem/1(Time)

== system Aenea_model/AUTOPILOTA/GESTIONE AUTOPILOTI1/Intervento Manager ==
  Manuale : Inport
  Ingaggio_AP : Inport  Port=2
  absE : Inport  Port=3
  absA : Inport  Port=4
  absT : Inport  Port=5
  Alarm_Timing_0.5sec : Subsystem
  Alarm_Timing_1sec : Subsystem
  Constant : Constant  Value=interventoE_1
  Constant1 : Constant  Value=interventoE_05
  Constant2 : Constant  Value=interventoT
  Constant3 : Constant  Value=interventoA_1
  Constant4 : Constant  Value=interventoA_05
  MATLAB Function1 : MATLAB Function  TreatAsAtomicUnit=on
  Switch : Switch  Criteria=u2 ~= 0
  Alarm_Intervento : Outport  VectorParamsAs1DForOutWhenUnconnected=off
  wires:
  Switch/1 -> Alarm_Intervento/1
  Manuale/1 -> MATLAB Function1/1(Manuale)
  Ingaggio_AP/1 -> MATLAB Function1/2(Ingaggio_AP)
  absE/1 -> MATLAB Function1/3(absE)
  absA/1 -> MATLAB Function1/4(absA)
  absT/1 -> MATLAB Function1/5(absT)
  MATLAB Function1/2(sw) -> Switch/2
  MATLAB Function1/1(Int_1) -> Alarm_Timing_1sec/1(Intervento_IN)
  MATLAB Function1/3(Int_05) -> Alarm_Timing_0.5sec/1(Intervento_IN)
  Alarm_Timing_1sec/1(Alarm) -> Switch/1
  Alarm_Timing_0.5sec/1(Alarm) -> Switch/3
  Constant/1 -> MATLAB Function1/6(interventoE_1)
  Constant1/1 -> MATLAB Function1/7(interventoE_05)
  Constant2/1 -> MATLAB Function1/10(interventoT)
  Constant3/1 -> MATLAB Function1/8(interventoA_1)
  Constant4/1 -> MATLAB Function1/9(interventoA_05)

== system Aenea_model/AUTOPILOTA/GESTIONE AUTOPILOTI1/Safe Manager ==
  note: Quando si preme il tasto Test SAFE MODE su QGC la Matlab Function riceve un valore di Veloc = 50 per due sec
      | e quindi per due sec essa restituisce Alarm_safe = 1. Dato che tale valore persiste per due secondi il Subsystem
      | successivo pone Alarm_Safe = 1. Esso successivamente è inviato allo state flow.
  Veloc : Inport
  phi : Inport  Port=2
  ingaggio_AP : Inport  Port=3
  Manuale : Inport  Port=4
  Alarm_Timing : Subsystem
  Constant : Constant  Value=safe_V
  Constant1 : Constant  Value=safe_phi
  MATLAB Function1 : MATLAB Function  TreatAsAtomicUnit=on
  Alarm_Safe : Outport  VectorParamsAs1DForOutWhenUnconnected=off
  wires:
  Alarm_Timing/1(Alarm) -> Alarm_Safe/1
  Veloc/1 -> MATLAB Function1/1(Veloc)
  ingaggio_AP/1 -> MATLAB Function1/3(ingaggio_AP)
  phi/1 -> MATLAB Function1/2(phi)
  MATLAB Function1/1(Alarm_safe) -> Alarm_Timing/1(Alarm_IN)
  Constant/1 -> MATLAB Function1/4(safe_V)
  Constant1/1 -> MATLAB Function1/5(safe_phi)
  Manuale/1 -> MATLAB Function1/6(Manuale)

== system Aenea_model/AUTOPILOTA/GESTIONE AUTOPILOTI1/abs comandi manuali ==
  comandi manuali : Inport
  Abs{,1..3} (4 alike) : Abs
  Bus Creator : BusCreator  Inputs=4
  Bus Selector : BusSelector  OutputSignals=Manual Elevator,Manual Aileron,Manual Rudder,Manual Throttle
  Out : Outport  VectorParamsAs1DForOutWhenUnconnected=off
  wires:
  comandi manuali/1 -> Bus Selector/1
  Bus Selector/1 -> Abs/1  "<Manual Elevator>"
  Abs/1 -> Bus Creator/1  "abs_Manual Elevator"
  Bus Selector/2 -> Abs1/1  "<Manual Aileron>"
  Bus Selector/3 -> Abs2/1  "<Manual Rudder>"
  Bus Selector/4 -> Abs3/1  "<Manual Throttle>"
  Abs1/1 -> Bus Creator/2  "abs_Manual Aileron"
  Abs2/1 -> Bus Creator/3  "abs_Manual Rudder"
  Abs3/1 -> Bus Creator/4  "abs_Manual Throttle"
  Bus Creator/1 -> Out/1

== system Aenea_model/AUTOPILOTA/Subsystem1/DECOLLO AUTOMATICO ==
  Tas : Inport
  h : Inport  Port=2
  modo : Inport  Port=3
  psi_imu : Inport  Port=4
  theta : Inport  Port=5
  V_ : Inport  Port=6
  Enable : EnablePort
  Chart1 : Stateflow chart  TreatAsAtomicUnit=on
  Memory : Memory
  Memory1 : Memory
  Radians to Degrees : simulink_extras/Transformations/Radians to Degrees
  Radians to Degrees1 : simulink_extras/Transformations/Radians to Degrees
  Sample and Hold : dspsigops/Sample and Hold  trig=Rising edge  initCond=0  latchinput=off
  Sample and Hold1 : dspsigops/Sample and Hold  trig=Rising edge  initCond=0  latchinput=off
  rotta_ATO : Outport  VectorParamsAs1DForOutWhenUnconnected=off
  Fase_ATO : Outport  Port=2  VectorParamsAs1DForOutWhenUnconnected=off
  manetta_ref_ATO : Outport  Port=3  VectorParamsAs1DForOutWhenUnconnected=off
  eq_rot_ATO : Outport  Port=4  VectorParamsAs1DForOutWhenUnconnected=off
  phi_ref_ATO : Outport  Port=5  VectorParamsAs1DForOutWhenUnconnected=off
  theta_ref_ATO : Outport  Port=6  VectorParamsAs1DForOutWhenUnconnected=off
  h_ref_ATO : Outport  Port=7  VectorParamsAs1DForOutWhenUnconnected=off
  Tas_ref_ATO : Outport  Port=8  VectorParamsAs1DForOutWhenUnconnected=off
  RC_ref_ATO : Outport  Port=9  VectorParamsAs1DForOutWhenUnconnected=off
  wires:
  Chart1/3(psi_ref) -> rotta_ATO/1  "ROTTA"
  modo/1 -> Chart1/1(modo)
  h/1 -> Chart1/3(h)
  Tas/1 -> Chart1/2(TAS)
  Chart1/10(psi_ref_selector) -> Memory/1
  Memory/1 -> Sample and Hold/Trigger
  Sample and Hold/1 -> Chart1/4(psi_hold)
  psi_imu/1 -> Radians to Degrees1/1
  Chart1/1(Fase_ATO) -> Fase_ATO/1
  Chart1/2(manetta_ref) -> manetta_ref_ATO/1
  Chart1/7(h_ref) -> h_ref_ATO/1
  Chart1/4(eq_rot) -> eq_rot_ATO/1
  Chart1/5(phi_ref) -> phi_ref_ATO/1
  Chart1/6(pitch_ref) -> theta_ref_ATO/1
  Chart1/8(Tas_ref) -> Tas_ref_ATO/1
  Chart1/9(RC_ref) -> RC_ref_ATO/1
  Sample and Hold1/1 -> Chart1/5(theta_ground_hold)
  Chart1/11(theta_ground_selector) -> Memory1/1
  Memory1/1 -> Sample and Hold1/Trigger
  theta/1 -> Radians to Degrees/1
  Radians to Degrees/1 -> Sample and Hold1/1
  V_/1 -> Chart1/6(V_)
  Radians to Degrees1/1 -> Sample and Hold/1

== system Aenea_model/AUTOPILOTA/Subsystem1/Subsystem ==
  In1 : Inport
  In2 : Inport  Port=2
  In3 : Inport  Port=3
  In4 : Inport  Port=4
  In5 : Inport  Port=5
  <IAS> : Inport  Port=6
  In7 : Inport  Port=7
  <ALT> : Inport  Port=8
  <HDG> : Inport  Port=9
  In10 : Inport  Port=10
  <RC> : Inport  Port=11
  In12 : Inport  Port=12
  <Ingaggio_AP> : Inport  Port=13
  In14 : Inport  Port=14
  Enable : EnablePort
  Abs : Abs
  Data Type Conversion{,1..3} (4 alike) : DataTypeConversion  OutDataTypeStr=double
  Memory{,1..3,6} (5 alike) : Memory  InheritSampleTime=on
  Radians to Degrees3 : simulink_extras/Transformations/Radians to Degrees
  VETTORIALE : MATLAB Function  TreatAsAtomicUnit=on
  Out1 : Outport  VectorParamsAs1DForOutWhenUnconnected=off
  Out2 : Outport  Port=2  VectorParamsAs1DForOutWhenUnconnected=off
  Out3 : Outport  Port=3  VectorParamsAs1DForOutWhenUnconnected=off
  Out4 : Outport  Port=4  VectorParamsAs1DForOutWhenUnconnected=off
  wires:
  Data Type Conversion1/1 -> VETTORIALE/8(VELOCITA)
  Memory1/1 -> VETTORIALE/18(ALT_pre)
  VETTORIALE/5(ingaggio_AP_mem) -> Memory6/1
  Data Type Conversion2/1 -> VETTORIALE/9(QUOTA)
  VETTORIALE/8(ALT_pre_mem) -> Memory1/1
  Radians to Degrees3/1 -> VETTORIALE/11(HEADING)
  Memory6/1 -> VETTORIALE/15(ingaggio_AP_pre)
  In12/1 -> VETTORIALE/13(h)
  Memory3/1 -> VETTORIALE/16(modo_pre)
  VETTORIALE/6(modo_pre_mem) -> Memory3/1
  Abs/1 -> VETTORIALE/10(RC)
  VETTORIALE/9(HDG_pre_mem) -> Memory/1
  Data Type Conversion3/1 -> Abs/1
  Memory/1 -> VETTORIALE/19(HDG_pre)
  Data Type Conversion/1 -> VETTORIALE/7(ROTTA)
  Memory2/1 -> VETTORIALE/17(IAS_pre)
  VETTORIALE/7(IAS_pre_mem) -> Memory2/1
  VETTORIALE/3(rotta_vett) -> Out3/1
  In1/1 -> VETTORIALE/1(modo)
  <ALT>/1 -> VETTORIALE/3(ALT)
  <RC>/1 -> VETTORIALE/5(I_RC)
  In5/1 -> Data Type Conversion3/1
  In4/1 -> Data Type Conversion2/1
  <Ingaggio_AP>/1 -> VETTORIALE/6(ingaggio_AP)
  In10/1 -> VETTORIALE/12(TAS)
  In7/1 -> Radians to Degrees3/1
  In3/1 -> Data Type Conversion1/1
  VETTORIALE/1(V_vett) -> Out1/1
  VETTORIALE/2(h_vett) -> Out2/1
  <IAS>/1 -> VETTORIALE/2(IAS)
  In2/1 -> Data Type Conversion/1
  In14/1 -> VETTORIALE/14(RC_default)
  VETTORIALE/4(RC_vett) -> Out4/1
  <HDG>/1 -> VETTORIALE/4(HDG)
